simulink model "RobotickyManipulator_Simscape"  (R2024a)
(part 2 of 3)

  Stojna_{5..8} (4 alike) : sm_lib/Body Elements/Brick Solid  BrickDimensions=[0.1 0.1 2]  BrickDimensionsUnits=m  ExportEntireGeometry=off  InertiaType=CalculateFromGeometry  BasedOnType=Density  Density=1000  DensityUnits=kg/m^3  Mass=1  MassUnits=kg  CenterOfMass=[0 0 0]  CenterOfMassUnits=m  MomentsOfInertia=[1 1 1]  MomentsOfInertiaUnits=kg*m^2  ProductsOfInertia=[0 0 0]  ProductsOfInertiaUnits=kg*m^2  GraphicType=FromGeometry  MarkerShape=Sphere  MarkerSize=10  GraphicVisPropType=SimpleVisualProperties  GraphicDiffuseColor=[0.4 0.4 0.4]  GraphicOpacity=1.0  GraphicSpecularColor=[0.5 0.5 0.5 1.0]  GraphicAmbientColor=[0.15 0.15 0.15 1.0]  GraphicEmissiveColor=[0.0 0.0 0.0 1.0]  GraphicShininess=75  DoExposeReferenceFrame=off  SerializedFrames=<Frames><Frame><Id>Frame2</Id><Value><Name>F2</Name><Origin><Source>GeometricFeature</Source><FeatureName>+z -x curve</FeatureName></Origin><PrimaryAxis><DefinedDirection>+Z</DefinedDirection><Source>ReferenceFrame</Source><SourceDirection>+Z</SourceDirection><FeatureName></FeatureName></PrimaryAxis><SecondaryAxis><DefinedDirection>+X</DefinedDirection><Source>ReferenceFrame</Source><SourceDirection>+X</SourceDirection><FeatureName></FeatureName></SecondaryAxis></Value></Frame></Frames>
  Stojny : Subsystem
  To Workspace1 : ToWorkspace  VariableName=nuzky1  SaveFormat=Structure With Time  SampleTime=-1
  To Workspace2 : ToWorkspace  VariableName=pohon1  SaveFormat=Structure With Time  SampleTime=-1
  To Workspace3 : ToWorkspace  VariableName=pohon2  SaveFormat=Structure With Time  SampleTime=-1
  To Workspace4 : ToWorkspace  VariableName=nuzky2  SaveFormat=Structure With Time  SampleTime=-1
  To Workspace5 : ToWorkspace  VariableName=nuzky3  SaveFormat=Structure With Time  SampleTime=-1
  To Workspace6 : ToWorkspace  VariableName=nuzky4  SaveFormat=Structure With Time  SampleTime=-1
  World Frame : sm_lib/Frames and Transforms/World Frame
  World Frame2 : sm_lib/Frames and Transforms/World Frame
  World Frame4 : sm_lib/Frames and Transforms/World Frame
  Zebrovani : Subsystem
  Zrychlení : Scope
  paralel : sm_lib/Body Elements/Brick Solid  BrickDimensions=[0.025 0.025 robot.delkaNuzek]  BrickDimensionsUnits=m  ExportEntireGeometry=off  InertiaType=CalculateFromGeometry  BasedOnType=Density  Density=1000  DensityUnits=kg/m^3  Mass=1  MassUnits=kg  CenterOfMass=[0 0 0]  CenterOfMassUnits=m  MomentsOfInertia=[1 1 1]  MomentsOfInertiaUnits=kg*m^2  ProductsOfInertia=[0 0 0]  ProductsOfInertiaUnits=kg*m^2  GraphicType=FromGeometry  MarkerShape=Sphere  MarkerSize=10  GraphicVisPropType=SimpleVisualProperties  GraphicDiffuseColor=[0.1 0.5 0.8]  GraphicOpacity=1.0  GraphicSpecularColor=[0.5 0.5 0.5 1.0]  GraphicAmbientColor=[0.15 0.15 0.15 1.0]  GraphicEmissiveColor=[0.0 0.0 0.0 1.0]  GraphicShininess=75  DoExposeReferenceFrame=off  SerializedFrames=<Frames><Frame><Id>Frame1</Id><Value><Name>F1</Name><Origin><Source>GeometricFeature</Source><FeatureName>+z surface</FeatureName></Origin><PrimaryAxis><DefinedDirection>+X</DefinedDirection><Source>ReferenceFrame</Source><SourceDirection>+Z</SourceDirection><FeatureName></FeatureName></PrimaryAxis><SecondaryAxis><DefinedDirection>+Z</DefinedDirection><Source>ReferenceFrame</Source><SourceDirection>+X</SourceDirection><FeatureName></FeatureName></SecondaryAxis></Value></Frame><Frame><Id>Frame2</Id><Value><Name>F2</Name><Origin><Source>GeometricFeature</Source><FeatureName>-z surface</FeatureName></Origin><PrimaryAxis><DefinedDirection>+Y</DefinedDirection><Source>ReferenceFrame</Source><SourceDirection>+Z</SourceDirection><FeatureName></FeatureName></PrimaryAxis><SecondaryAxis><DefinedDirection>+Z</DefinedDirection><Source>ReferenceFrame</Source><SourceDirection>+X</SourceDirection><FeatureName></FeatureName></SecondaryAxis></Value></Frame></Frames>
  paralel.11 : sm_lib/Body Elements/Brick Solid  BrickDimensions=[0.025 0.025 robot.delkaNuzek]  BrickDimensionsUnits=m  ExportEntireGeometry=off  InertiaType=CalculateFromGeometry  BasedOnType=Density  Density=1000  DensityUnits=kg/m^3  Mass=1  MassUnits=kg  CenterOfMass=[0 0 0]  CenterOfMassUnits=m  MomentsOfInertia=[1 1 1]  MomentsOfInertiaUnits=kg*m^2  ProductsOfInertia=[0 0 0]  ProductsOfInertiaUnits=kg*m^2  GraphicType=FromGeometry  MarkerShape=Sphere  MarkerSize=10  GraphicVisPropType=SimpleVisualProperties  GraphicDiffuseColor=[0.1 0.5 0.8]  GraphicOpacity=1.0  GraphicSpecularColor=[0.5 0.5 0.5 1.0]  GraphicAmbientColor=[0.15 0.15 0.15 1.0]  GraphicEmissiveColor=[0.0 0.0 0.0 1.0]  GraphicShininess=75  DoExposeReferenceFrame=off  SerializedFrames=<Frames><Frame><Id>Frame1</Id><Value><Name>F1</Name><Origin><Source>GeometricFeature</Source><FeatureName>+z surface</FeatureName></Origin><PrimaryAxis><DefinedDirection>+X</DefinedDirection><Source>ReferenceFrame</Source><SourceDirection>+Z</SourceDirection><FeatureName></FeatureName></PrimaryAxis><SecondaryAxis><DefinedDirection>+Z</DefinedDirection><Source>ReferenceFrame</Source><SourceDirection>+X</SourceDirection><FeatureName></FeatureName></SecondaryAxis></Value></Frame><Frame><Id>Frame2</Id><Value><Name>F2</Name><Origin><Source>GeometricFeature</Source><FeatureName>-z surface</FeatureName></Origin><PrimaryAxis><DefinedDirection>+Y</DefinedDirection><Source>ReferenceFrame</Source><SourceDirection>+Z</SourceDirection><FeatureName></FeatureName></PrimaryAxis><SecondaryAxis><DefinedDirection>+Z</DefinedDirection><Source>ReferenceFrame</Source><SourceDirection>+X</SourceDirection><FeatureName></FeatureName></SecondaryAxis></Value></Frame></Frames>
  paralel.12 : sm_lib/Body Elements/Brick Solid  BrickDimensions=[0.05 0.1 robot.delkaNuzek]  BrickDimensionsUnits=m  ExportEntireGeometry=off  InertiaType=CalculateFromGeometry  BasedOnType=Density  Density=1000  DensityUnits=kg/m^3  Mass=1  MassUnits=kg  CenterOfMass=[0 0 0]  CenterOfMassUnits=m  MomentsOfInertia=[1 1 1]  MomentsOfInertiaUnits=kg*m^2  ProductsOfInertia=[0 0 0]  ProductsOfInertiaUnits=kg*m^2  GraphicType=FromGeometry  MarkerShape=Sphere  MarkerSize=10  GraphicVisPropType=SimpleVisualProperties  GraphicDiffuseColor=[0.1 0.5 0.8]  GraphicOpacity=1.0  GraphicSpecularColor=[0.5 0.5 0.5 1.0]  GraphicAmbientColor=[0.15 0.15 0.15 1.0]  GraphicEmissiveColor=[0.0 0.0 0.0 1.0]  GraphicShininess=75  DoExposeReferenceFrame=off  SerializedFrames=<Frames><Frame><Id>Frame1</Id><Value><Name>F1</Name><Origin><Source>GeometricFeature</Source><FeatureName>+z surface</FeatureName></Origin><PrimaryAxis><DefinedDirection>+X</DefinedDirection><Source>ReferenceFrame</Source><SourceDirection>+Z</SourceDirection><FeatureName></FeatureName></PrimaryAxis><SecondaryAxis><DefinedDirection>+Z</DefinedDirection><Source>ReferenceFrame</Source><SourceDirection>+X</SourceDirection><FeatureName></FeatureName></SecondaryAxis></Value></Frame><Frame><Id>Frame2</Id><Value><Name>F2</Name><Origin><Source>GeometricFeature</Source><FeatureName>-z surface</FeatureName></Origin><PrimaryAxis><DefinedDirection>+Y</DefinedDirection><Source>ReferenceFrame</Source><SourceDirection>+Z</SourceDirection><FeatureName></FeatureName></PrimaryAxis><SecondaryAxis><DefinedDirection>+Z</DefinedDirection><Source>ReferenceFrame</Source><SourceDirection>+X</SourceDirection><FeatureName></FeatureName></SecondaryAxis></Value></Frame></Frames>
  paralel.13 : sm_lib/Body Elements/Brick Solid  BrickDimensions=[0.025 0.025 robot.delkaNuzek]  BrickDimensionsUnits=m  ExportEntireGeometry=off  InertiaType=CalculateFromGeometry  BasedOnType=Density  Density=1000  DensityUnits=kg/m^3  Mass=1  MassUnits=kg  CenterOfMass=[0 0 0]  CenterOfMassUnits=m  MomentsOfInertia=[1 1 1]  MomentsOfInertiaUnits=kg*m^2  ProductsOfInertia=[0 0 0]  ProductsOfInertiaUnits=kg*m^2  GraphicType=FromGeometry  MarkerShape=Sphere  MarkerSize=10  GraphicVisPropType=SimpleVisualProperties  GraphicDiffuseColor=[0.1 0.5 0.8]  GraphicOpacity=1.0  GraphicSpecularColor=[0.5 0.5 0.5 1.0]  GraphicAmbientColor=[0.15 0.15 0.15 1.0]  GraphicEmissiveColor=[0.0 0.0 0.0 1.0]  GraphicShininess=75  DoExposeReferenceFrame=off  SerializedFrames=<Frames><Frame><Id>Frame1</Id><Value><Name>F1</Name><Origin><Source>GeometricFeature</Source><FeatureName>+z surface</FeatureName></Origin><PrimaryAxis><DefinedDirection>+X</DefinedDirection><Source>ReferenceFrame</Source><SourceDirection>+Z</SourceDirection><FeatureName></FeatureName></PrimaryAxis><SecondaryAxis><DefinedDirection>+Z</DefinedDirection><Source>ReferenceFrame</Source><SourceDirection>+X</SourceDirection><FeatureName></FeatureName></SecondaryAxis></Value></Frame><Frame><Id>Frame2</Id><Value><Name>F2</Name><Origin><Source>GeometricFeature</Source><FeatureName>-z surface</FeatureName></Origin><PrimaryAxis><DefinedDirection>+Y</DefinedDirection><Source>ReferenceFrame</Source><SourceDirection>+Z</SourceDirection><FeatureName></FeatureName></PrimaryAxis><SecondaryAxis><DefinedDirection>+Z</DefinedDirection><Source>ReferenceFrame</Source><SourceDirection>+X</SourceDirection><FeatureName></FeatureName></SecondaryAxis></Value></Frame></Frames>
  paralel.14 : sm_lib/Body Elements/Brick Solid  BrickDimensions=[0.025 0.025 robot.delkaNuzek]  BrickDimensionsUnits=m  ExportEntireGeometry=off  InertiaType=CalculateFromGeometry  BasedOnType=Density  Density=1000  DensityUnits=kg/m^3  Mass=1  MassUnits=kg  CenterOfMass=[0 0 0]  CenterOfMassUnits=m  MomentsOfInertia=[1 1 1]  MomentsOfInertiaUnits=kg*m^2  ProductsOfInertia=[0 0 0]  ProductsOfInertiaUnits=kg*m^2  GraphicType=FromGeometry  MarkerShape=Sphere  MarkerSize=10  GraphicVisPropType=SimpleVisualProperties  GraphicDiffuseColor=[0.1 0.5 0.8]  GraphicOpacity=1.0  GraphicSpecularColor=[0.5 0.5 0.5 1.0]  GraphicAmbientColor=[0.15 0.15 0.15 1.0]  GraphicEmissiveColor=[0.0 0.0 0.0 1.0]  GraphicShininess=75  DoExposeReferenceFrame=off  SerializedFrames=<Frames><Frame><Id>Frame1</Id><Value><Name>F1</Name><Origin><Source>GeometricFeature</Source><FeatureName>+z surface</FeatureName></Origin><PrimaryAxis><DefinedDirection>+X</DefinedDirection><Source>ReferenceFrame</Source><SourceDirection>+Z</SourceDirection><FeatureName></FeatureName></PrimaryAxis><SecondaryAxis><DefinedDirection>+Z</DefinedDirection><Source>ReferenceFrame</Source><SourceDirection>+X</SourceDirection><FeatureName></FeatureName></SecondaryAxis></Value></Frame><Frame><Id>Frame2</Id><Value><Name>F2</Name><Origin><Source>GeometricFeature</Source><FeatureName>-z surface</FeatureName></Origin><PrimaryAxis><DefinedDirection>+Y</DefinedDirection><Source>ReferenceFrame</Source><SourceDirection>+Z</SourceDirection><FeatureName></FeatureName></PrimaryAxis><SecondaryAxis><DefinedDirection>+Z</DefinedDirection><Source>ReferenceFrame</Source><SourceDirection>+X</SourceDirection><FeatureName></FeatureName></SecondaryAxis></Value></Frame></Frames>
  paralel.9 : sm_lib/Body Elements/Brick Solid  BrickDimensions=[0.05 0.1 robot.delkaNuzek]  BrickDimensionsUnits=m  ExportEntireGeometry=off  InertiaType=CalculateFromGeometry  BasedOnType=Density  Density=1000  DensityUnits=kg/m^3  Mass=1  MassUnits=kg  CenterOfMass=[0 0 0]  CenterOfMassUnits=m  MomentsOfInertia=[1 1 1]  MomentsOfInertiaUnits=kg*m^2  ProductsOfInertia=[0 0 0]  ProductsOfInertiaUnits=kg*m^2  GraphicType=FromGeometry  MarkerShape=Sphere  MarkerSize=10  GraphicVisPropType=SimpleVisualProperties  GraphicDiffuseColor=[0.1 0.5 0.8]  GraphicOpacity=1.0  GraphicSpecularColor=[0.5 0.5 0.5 1.0]  GraphicAmbientColor=[0.15 0.15 0.15 1.0]  GraphicEmissiveColor=[0.0 0.0 0.0 1.0]  GraphicShininess=75  DoExposeReferenceFrame=off  SerializedFrames=<Frames><Frame><Id>Frame1</Id><Value><Name>F1</Name><Origin><Source>GeometricFeature</Source><FeatureName>+z surface</FeatureName></Origin><PrimaryAxis><DefinedDirection>+X</DefinedDirection><Source>ReferenceFrame</Source><SourceDirection>+Z</SourceDirection><FeatureName></FeatureName></PrimaryAxis><SecondaryAxis><DefinedDirection>+Z</DefinedDirection><Source>ReferenceFrame</Source><SourceDirection>+X</SourceDirection><FeatureName></FeatureName></SecondaryAxis></Value></Frame><Frame><Id>Frame2</Id><Value><Name>F2</Name><Origin><Source>GeometricFeature</Source><FeatureName>-z surface</FeatureName></Origin><PrimaryAxis><DefinedDirection>+Y</DefinedDirection><Source>ReferenceFrame</Source><SourceDirection>+Z</SourceDirection><FeatureName></FeatureName></PrimaryAxis><SecondaryAxis><DefinedDirection>+Z</DefinedDirection><Source>ReferenceFrame</Source><SourceDirection>+X</SourceDirection><FeatureName></FeatureName></SecondaryAxis></Value></Frame></Frames>
  pricny_nosnik : sm_lib/Body Elements/Brick Solid  BrickDimensions=[0.1 robot.sirka_y-0.3 0.2]  BrickDimensionsUnits=m  ExportEntireGeometry=off  InertiaType=CalculateFromGeometry  BasedOnType=Density  Density=1000  DensityUnits=kg/m^3  Mass=1  MassUnits=kg  CenterOfMass=[0 0 0]  CenterOfMassUnits=m  MomentsOfInertia=[1 1 1]  MomentsOfInertiaUnits=kg*m^2  ProductsOfInertia=[0 0 0]  ProductsOfInertiaUnits=kg*m^2  GraphicType=FromGeometry  MarkerShape=Sphere  MarkerSize=10  GraphicVisPropType=SimpleVisualProperties  GraphicDiffuseColor=[0.4 0.4 0.4]  GraphicOpacity=1.0  GraphicSpecularColor=[0.5 0.5 0.5 1.0]  GraphicAmbientColor=[0.15 0.15 0.15 1.0]  GraphicEmissiveColor=[0.0 0.0 0.0 1.0]  GraphicShininess=75  DoExposeReferenceFrame=off  SerializedFrames=<Frames><Frame><Id>Frame1</Id><Value><Name>+y</Name><Origin><Source>GeometricFeature</Source><FeatureName>-x -y curve</FeatureName></Origin><PrimaryAxis><DefinedDirection>+Z</DefinedDirection><Source>ReferenceFrame</Source><SourceDirection>+Z</SourceDirection><FeatureName></FeatureName></PrimaryAxis><SecondaryAxis><DefinedDirection>+X</DefinedDirection><Source>ReferenceFrame</Source><SourceDirection>+X</SourceDirection><FeatureName></FeatureName></SecondaryAxis></Value></Frame><Frame><Id>Frame2</Id><Value><Name>F2</Name><Origin><Source>GeometricFeature</Source><FeatureName>-y +z curve</FeatureName></Origin><PrimaryAxis><DefinedDirection>+Z</DefinedDirection><Source>ReferenceFrame</Source><SourceDirection>+Z</SourceDirection><FeatureName></FeatureName></PrimaryAxis><SecondaryAxis><DefinedDirection>+X</DefinedDirection><Source>ReferenceFrame</Source><SourceDirection>+X</SourceDirection><FeatureName></FeatureName></SecondaryAxis></Value></Frame></Frames>
  wires:
  Constant10/1 -> Simulink-PS Converter13/1
  Constant1/1 -> Simulink-PS Converter1/1
  Constant8/1 -> Simulink-PS Converter11/1
  Constant2/1 -> Simulink-PS Converter2/1
  Constant3/1 -> Simulink-PS Converter3/1
  Constant4/1 -> Simulink-PS Converter4/1
  Constant6/1 -> Simulink-PS Converter10/1
  Constant5/1 -> Simulink-PS Converter6/1
  PS-Simulink Converter10/1 -> To Workspace4/1
  PS-Simulink Converter11/1 -> To Workspace5/1
  PS-Simulink Converter12/1 -> To Workspace6/1
  PS-Simulink Converter1/1 -> To Workspace1/1
  From Workspace8/1 -> Simulink-PS Converter5/1
  PS-Simulink Converter2/1 -> Mux/1  "vz"
  PS-Simulink Converter6/1 -> Mux1/2  "ay"
  From Workspace7/1 -> Simulink-PS Converter9/1
  From Workspace5/1 -> Simulink-PS Converter7/1
  Mux1/1 -> Zrychlení/1
  PS-Simulink Converter14/1 -> Mux1/4  "bz"
  From Workspace6/1 -> Simulink-PS Converter8/1
  PS-Simulink Converter13/1 -> Mux/4  "wx"
  PS-Simulink Converter4/1 -> Mux/3  "vx"
  PS-Simulink Converter3/1 -> Mux/2  "vy"
  PS-Simulink Converter5/1 -> Mux1/1  "az"
  Mux/1 -> Rychlosti/1
  PS-Simulink Converter7/1 -> Mux1/3  "ax"
  PS-Simulink Converter9/1 -> To Workspace3/1
  PS-Simulink Converter8/1 -> To Workspace2/1
  connections:
  Simulink-PS Converter13/RConn1 -- Prismatic Joint4/LConn2
  Prismatic Joint4/RConn1 -- Rigid Transform45/LConn1
  Cylindrical Solid24/LConn1 -- Rigid Transform54/RConn1
  Simulink-PS Converter6/RConn1 -- Prismatic Joint1/LConn2
  Cylindrical Solid22/LConn1 -- Rigid Transform51/RConn1
  Prismatic Joint4/LConn1 -- Rigid Transform44/RConn1
  Cylindrical Solid15/RConn1 -- Revolute Joint3/LConn1
  Rigid Transform60/RConn1 -- Brick Solid19/RConn1
  Cylindrical Solid18/RConn1 -- Cylindrical Solid19/RConn1
  Cylindrical Solid25/RConn1 -- Cylindrical Solid30/RConn1
  Cylindrical Solid23/RConn1 -- Cylindrical Solid32/RConn1
  Cylindrical Solid26/RConn1 -- Cylindrical Solid31/RConn1
  Cylindrical Solid40/LConn1 -- Rigid Transform59/RConn1
  Simulink-PS Converter10/RConn1 -- Prismatic Joint2/LConn2
  Rigid Transform35/RConn1 -- Cylindrical Solid15/LConn1
  Rigid Transform46/RConn1 -- Brick Solid17/RConn1
  Rigid Transform36/LConn1 -- Brick Solid6/RConn1
  Cylindrical Solid35/LConn1 -- Rigid Transform48/RConn1
  Cylindrical Solid30/LConn1 -- Rigid Transform55/RConn1
  Cylindrical Solid21/RConn1 -- Cylindrical Solid22/RConn1
  Cylindrical Solid20/RConn1 -- Cylindrical Solid35/RConn1
  Cylindrical Solid28/LConn1 -- Rigid Transform57/RConn1
  Prismatic Joint3/LConn1 -- Rigid Transform42/RConn1
  Cylindrical Solid17/LConn1 -- Rigid Transform41/RConn1
  Simulink-PS Converter2/RConn1 -- Revolute Joint2/LConn2
  Cylindrical Solid19/LConn1 -- Rigid Transform47/RConn1
  Brick Solid11/LConn1 -- Revolute Joint2/RConn1
  Cylindrical Solid/RConn1 -- Cylindrical Solid24/RConn1
  Revolute Joint2/LConn1 -- Cylindrical Solid16/RConn1
  Brick Solid13/RConn1 -- Rigid Transform44/LConn1
  Cylindrical Solid31/LConn1 -- Rigid Transform56/RConn1
  Cylindrical Solid36/RConn1 -- Cylindrical Solid37/RConn1
  Cylindrical Solid14/RConn1 -- Revolute Joint4/LConn1
  Cylindrical Solid37/LConn1 -- Rigid Transform49/RConn1
  Cylindrical Solid32/LConn1 -- Rigid Transform52/RConn1
  Prismatic Joint2/RConn1 -- Rigid Transform39/LConn1
  Cylindrical Solid14/LConn1 -- Rigid Transform29/RConn1
  Cylindrical Solid27/RConn1 -- Cylindrical Solid28/RConn1
  Cylindrical Solid16/LConn1 -- Rigid Transform40/RConn1
  Prismatic Joint1/RConn1 -- Rigid Transform37/LConn1
  Cylindrical Solid39/RConn1 -- Cylindrical Solid40/RConn1
  Prismatic Joint2/LConn1 -- Rigid Transform38/RConn1
  Simulink-PS Converter11/RConn1 -- Prismatic Joint3/LConn2
  Brick Solid11/RConn1 -- Rigid Transform42/LConn1
  Brick Solid13/LConn1 -- Revolute Joint1/RConn1
  Cylindrical Solid33/RConn1 -- Cylindrical Solid34/RConn1
  Brick Solid4/RConn1 -- Rigid Transform38/LConn1
  Simulink-PS Converter3/RConn1 -- Revolute Joint3/LConn2
  Cylindrical Solid29/RConn1 -- Cylindrical Solid38/RConn1
  Rigid Transform61/RConn1 -- Brick Solid20/RConn1
  Rigid Transform54/LConn1 -- Rigid Transform55/LConn1 -- Rigid Transform56/LConn1 -- Brick Solid5/RConn1 -- Rigid Transform60/LConn1 -- Rigid Transform39/RConn1
  Revolute Joint1/LConn1 -- Cylindrical Solid17/RConn1
  Brick Solid6/LConn1 -- Revolute Joint3/RConn1
  Rigid Transform59/LConn1 -- Rigid Transform57/LConn1 -- Rigid Transform58/LConn1 -- Rigid Transform61/LConn1 -- Rigid Transform37/RConn1 -- Brick Solid1/RConn1
  Rigid Transform53/LConn1 -- Rigid Transform52/LConn1 -- Rigid Transform51/LConn1 -- Rigid Transform50/LConn1 -- Rigid Transform43/RConn1 -- Brick Solid12/RConn1
  Cylindrical Solid38/LConn1 -- Rigid Transform58/RConn1
  Cylindrical Solid34/LConn1 -- Rigid Transform53/RConn1
  Simulink-PS Converter4/RConn1 -- Revolute Joint4/LConn2
  Rigid Transform50/RConn1 -- Brick Solid18/RConn1
  Rigid Transform45/RConn1 -- Rigid Transform46/LConn1 -- Rigid Transform48/LConn1 -- Rigid Transform47/LConn1 -- Rigid Transform49/LConn1 -- Brick Solid16/RConn1
  Simulink-PS Converter1/RConn1 -- Revolute Joint1/LConn2
  Prismatic Joint3/RConn1 -- Rigid Transform43/LConn1
  Brick Solid4/LConn1 -- Revolute Joint4/RConn1
  Prismatic Joint1/LConn1 -- Rigid Transform36/RConn1
  Brick Solid7/RConn4 -- Rigid Transform35/LConn1
  Brick Solid7/LConn4 -- Rigid Transform29/LConn1
  Brick Solid7/LConn3 -- Rigid Transform62/LConn1
  Rigid Transform40/LConn1 -- Brick Solid7/LConn5
  Cylindrical Solid2/RConn1 -- paralel.11/LConn1
  PS-Simulink Converter11/LConn1 -- Revolute Joint25/RConn2
  Cylindrical Solid12/LConn1 -- Revolute Joint24/RConn1
  Cylindrical Solid2/LConn1 -- Revolute Joint26/RConn1
  Revolute Joint30/RConn1 -- Brick Solid15/RConn1
  Revolute Joint24/LConn1 -- paralel.14/RConn1
  Brick Solid7/RConn1 -- Brick Solid3/RConn5
  Pohon4/LConn1 -- Rigid Transform23/RConn1
  Cylindrical Solid9/LConn1 -- Brick Solid15/RConn2
  Brick Solid3/LConn3 -- Prismatic Joint/RConn1
  Cylindrical Solid5/LConn1 -- paralel/RConn1
  Cylindrical Solid1/LConn1 -- Revolute Joint21/RConn1
  Revolute Joint31/LConn1 -- Cylindrical Solid10/RConn1
  Cylindrical Solid12/RConn1 -- Brick Solid3/LConn2
  Cylindrical Solid7/LConn1 -- paralel.11/RConn1
  Brick Solid3/RConn1 -- Belt-Cable End2/LConn1
  Revolute Joint25/RConn1 -- paralel.12/LConn1
  Rigid Transform41/LConn1 -- Brick Solid7/RConn3
  Cylindrical Solid13/RConn1 -- Brick Solid3/RConn2
  Revolute Joint20/RConn1 -- Cylindrical Solid3/LConn1
  PS-Simulink Converter1/LConn1 -- Revolute Joint20/RConn2
  Cylindrical Solid7/RConn1 -- Revolute Joint30/LConn1
  Cylindrical Solid13/LConn1 -- Revolute Joint22/RConn1
  Revolute Joint31/RConn1 -- paralel.14/LConn1
  Revolute Joint22/LConn1 -- paralel.12/RConn1
  Belt-Cable End2/RConn1 -- Belt-Cable Properties2/LConn1 -- Belt-Cable Spool2/RConn1
  Cylindrical Solid4/LConn1 -- paralel.9/RConn1
  Cylindrical Solid6/RConn1 -- Revolute Joint25/LConn1
  Brick Solid8/RConn1 -- Brick Solid15/LConn4
  Prismatic Joint/LConn1 -- Brick Solid14/LConn3
  Revolute Joint28/RConn1 -- Brick Solid15/LConn2
  Cylindrical Solid11/LConn1 -- Revolute Joint23/RConn1
  paralel.13/RConn1 -- Revolute Joint23/LConn1
  Cylindrical Solid3/RConn1 -- paralel.9/LConn1
  Rigid Transform23/LConn1 -- Revolute Joint32/RConn1 -- Rigid Transform24/LConn1
  Cylindrical Solid5/RConn1 -- Revolute Joint29/LConn1
  Revolute Joint27/RConn1 -- paralel.13/LConn1
  Revolute Joint26/LConn1 -- Brick Solid14/LConn2
  PS-Simulink Converter12/LConn1 -- Revolute Joint22/RConn2
  PS-Simulink Converter10/LConn1 -- Revolute Joint28/RConn2
  Cylindrical Solid4/RConn1 -- Revolute Joint28/LConn1
  Cylindrical Solid8/LConn1 -- Belt-Cable Spool2/LConn1
  Revolute Joint21/LConn1 -- Brick Solid14/LConn1
  Cylindrical Solid10/LConn1 -- Brick Solid15/LConn3
  Cylindrical Solid1/RConn1 -- paralel/LConn1
  Cylindrical Solid11/RConn1 -- Brick Solid3/LConn1
  Cylindrical Solid9/RConn1 -- Revolute Joint27/LConn1
  Pohon4/RConn1 -- Cylindrical Solid8/RConn1
  Revolute Joint29/RConn1 -- Brick Solid15/LConn1
  Brick Solid14/RConn2 -- Revolute Joint20/LConn1
  Brick Solid14/RConn1 -- Rigid Transform24/RConn1
  Cylindrical Solid6/LConn1 -- Brick Solid15/RConn3
  PS-Simulink Converter14/LConn1 -- Bushing Joint/RConn9
  PS-Simulink Converter7/LConn1 -- Bushing Joint/RConn3
  Simulink-PS Converter7/RConn1 -- Bushing Joint/LConn2
  Simulink-PS Converter9/RConn1 -- Bushing Joint/LConn4
  Simulink-PS Converter8/RConn1 -- Bushing Joint/LConn3
  Simulink-PS Converter5/RConn1 -- Bushing Joint/LConn5
  Bushing Joint/RConn8 -- PS-Simulink Converter13/LConn1
  Bushing Joint/LConn1 -- World Frame4/RConn1
  PS-Simulink Converter4/LConn1 -- Bushing Joint/RConn2
  PS-Simulink Converter6/LConn1 -- Bushing Joint/RConn5
  PS-Simulink Converter3/LConn1 -- Bushing Joint/RConn4
  PS-Simulink Converter2/LConn1 -- Bushing Joint/RConn6
  PS-Simulink Converter5/LConn1 -- Bushing Joint/RConn7
  Rigid Transform62/RConn1 -- Bushing Joint/RConn1 -- Rigid/LConn1
  Kocka/LConn3 -- Revolute Joint32/LConn1
  Rigid Transform33/RConn1 -- Stojna_7/LConn1
  Brick Solid10/LConn3 -- Příčný nosník5/LConn1
  Rigid Transform33/LConn1 -- Stojna_2/LConn2
  Rigid Transform5/LConn1 -- Příčný nosník/LConn2
  Rigid Transform2/RConn1 -- Pohon/RConn1
  Rigid Transform31/RConn1 -- Stojna_5/LConn1
  Rigid Transform5/RConn1 -- Pohon2/LConn1
  Stojna_1/RConn1 -- Podélný nosník_1/LConn1
  Rigid Transform34/LConn1 -- Stojna_1/LConn2
  Rigid Transform22/RConn1 -- Stojna_2/RConn1
  Rigid Transform31/LConn1 -- Stojna_4/RConn1
  Rigid Transform6/RConn1 -- pricny_nosnik/LConn1
  Příčný nosník4/LConn1 -- Rigid Transform/RConn1
  PS-Simulink Converter9/LConn1 -- Pohon2/RConn2
  Brick Solid10/RConn2 -- Rigid Transform6/LConn1
  Rigid Transform1/LConn1 -- Podélný nosník_1/LConn2
  Brick Solid9/LConn1 -- Příčný nosník/LConn1
  Rigid Transform/LConn1 -- Brick Solid10/LConn2
  Podélný nosník_1/RConn1 -- Stojna_4/LConn1
  Pohon2/RConn1 -- Rigid Transform4/RConn1
  Rigid Transform2/LConn1 -- Brick Solid2/LConn2
  Brick Solid/RConn1 -- Rigid Transform7/LConn1
  Rigid Transform32/RConn1 -- Stojna_6/LConn1
  Stojna_2/LConn1 -- Příčný nosník1/LConn1 -- Brick Solid2/LConn1
  Brick Solid10/RConn1 -- Rigid Transform3/LConn1
  Brick Solid10/LConn1 -- Příčný nosník/RConn1
  Rigid Transform32/LConn1 -- Stojna_3/RConn1
  Rigid Transform 190/RConn1 -- Pohon1/RConn1
  Rigid Transform34/RConn1 -- Stojna_8/LConn1
  Solver Configuration/RConn1 -- Rigid Transform25/RConn1 -- Stojna_1/LConn1 -- Mechanism Configuration/RConn1
  Kocka/RConn2 -- Rigid Transform4/LConn1
  Rigid Transform3/RConn1 -- Pohon/LConn1
  Brick Solid9/RConn1 -- Rigid Transform 190/LConn1
  World Frame2/RConn1 -- Rigid Stojny/LConn1 -- Rigid Transform22/LConn1
  Rigid Transform1/RConn1 -- Pohon1/LConn1
  Brick Solid2/RConn1 -- Stojna_3/LConn1 -- Příčný nosník2/LConn1
  PS-Simulink Converter8/LConn1 -- Pohon1/RConn2
  Zebrovani/LConn1 -- pricny_nosnik/RConn1
  Stojny/LConn1 -- Rigid Stojny/RConn1
  Rigid Transform7/RConn1 -- Rigid Transform25/LConn1 -- R1/LConn1 -- R2/LConn1 -- R3/LConn1 -- R4/LConn1 -- R5/LConn1 -- R6/LConn1 -- R7/LConn1 -- R8/LConn1 -- R9/LConn1 -- R10/LConn1 -- R11/LConn1 -- World Frame/RConn1 -- R12/LConn1
  S2/RConn1 -- R2/RConn1
  S4/RConn1 -- R4/RConn1
  S5/RConn1 -- R5/RConn1
  S6/RConn1 -- R6/RConn1
  S7/RConn1 -- R7/RConn1
  S8/RConn1 -- R8/RConn1
  S9/RConn1 -- R9/RConn1
  S10/RConn1 -- R10/RConn1
  S11/RConn1 -- R11/RConn1
  S12/RConn1 -- R12/RConn1
  S3/RConn1 -- R3/RConn1
  S1/RConn1 -- R1/RConn1
